simulink model "q1"  (R2025a)
settings: Solver=VariableStepAuto  StartTime=0.0  StopTime=90  RelTol=1e-3
settings Model: Creator=dtemu  LastModifiedBy=dtemu

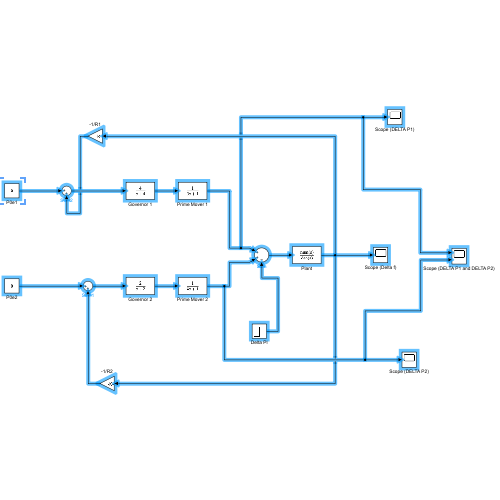
[thumbnail: Simulink's stored preview of the top-level diagram]
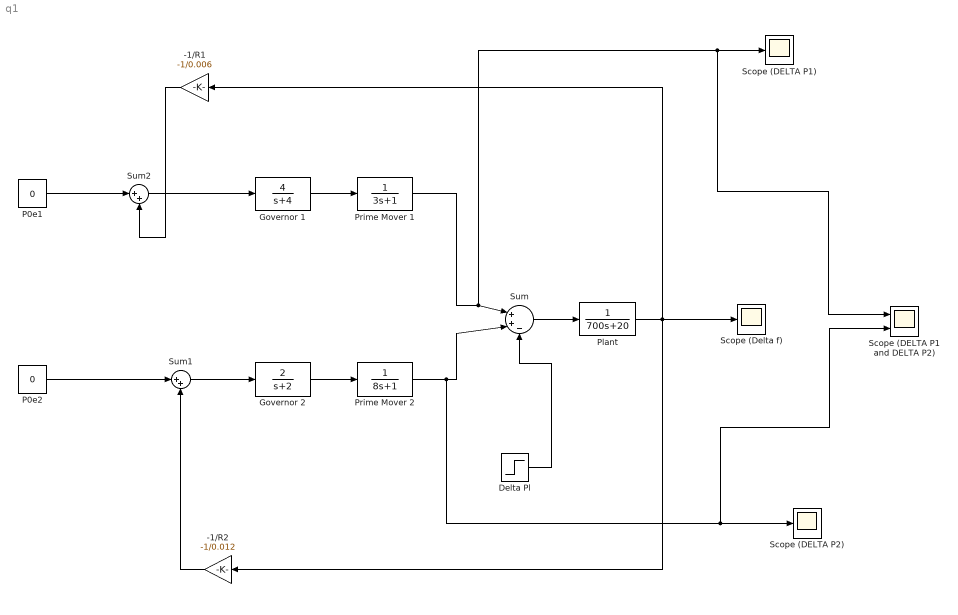
== system q1 ==
  -1/R1 : Gain  Gain=-1/0.006
  -1/R2 : Gain  Gain=-1/0.012
  Delta Pl : Step  Time=0  After=100  SampleTime=0
  Governor 1 : TransferFcn  Numerator=[4]  Denominator=[1 4]
  Governor 2 : TransferFcn  Numerator=[2]  Denominator=[1 2]
  P0e1 : Constant  Value=0
  P0e2 : Constant  Value=0
  Plant : TransferFcn  Denominator=[700 20]
  Prime Mover 1 : TransferFcn  Denominator=[3 1]
  Prime Mover 2 : TransferFcn  Denominator=[8 1]
  Scope (DELTA P1 and DELTA P2) : Scope  NumInputPorts=2
      settings: ActiveDisplayYMinimum=-8.8695692864813225  ActiveDisplayYMaximum=96.562935220846214  DataLoggingVariableName=ScopeData3
  Scope (DELTA P1) : Scope
      settings: ActiveDisplayYMinimum=-8.8695692864813225  ActiveDisplayYMaximum=96.562935220846214  DataLoggingVariableName=ScopeData2
  Scope (DELTA P2) : Scope
      settings: ActiveDisplayYMinimum=-3.8120262778400225  ActiveDisplayYMaximum=35.413493005363385
  Scope (Delta f) : Scope
      settings: ActiveDisplayYMinimum=-3.6930002436648017  ActiveDisplayYMaximum=2.1031707674875122
  Sum : Sum  Inputs=|++-
  Sum1 : Sum  Inputs=|++
  Sum2 : Sum  Inputs=|++
  wires:
  Delta Pl/1 -> Sum/3
  Governor 1/1 -> Prime Mover 1/1
  Governor 2/1 -> Prime Mover 2/1
  Prime Mover 2/1 -> Scope (DELTA P1 and DELTA P2)/2, Scope (DELTA P2)/1, Sum/2
  Plant/1 -> -1/R1/1, Scope (Delta f)/1, -1/R2/1
  -1/R2/1 -> Sum1/2
  Sum1/1 -> Governor 2/1
  -1/R1/1 -> Sum2/2
  Sum2/1 -> Governor 1/1
  P0e1/1 -> Sum2/1
  P0e2/1 -> Sum1/1
  Sum/1 -> Plant/1
  Prime Mover 1/1 -> Scope (DELTA P1 and DELTA P2)/1, Scope (DELTA P1)/1, Sum/1
